simulink library "Display_THB3"  (Simulink 8.2)
settings: Solver=ode45  StartTime=0.0  StopTime=10.0  RelTol=1e-3
libraries: carnot x3
settings Model: Creator=lena.frank  LastModifiedBy=drhf

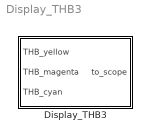
== system Display_THB3 ==
  Display_THB3 : Subsystem  mask(display THB){t=on, m=off, p=off, id=off, mix=off, d=off}
      mask prompts: t "temperature [degree centigrade]"; m "massflow [kg/s]"; p "pressure [Pa]"; id "fluid ID (1 = water, 2 = air, 3 = cotton oil, 4 = water-glycol)"; mix "fluid mix"; d "diameter [m]"
      mask help: Displays the ticked values from four THB.
      mask init:
      | v=[];
      | if (t)
      |     v  = [2];
      | end
      | if (m)
      |     v= [v 3];
      | end
      | if (p)
      |     v = [v 4];
      | end
      | if (id)
      |     v = [v 5];
      | end
      | if (mix)
      |     v = [v 6];
      | end
      | if (d)
      |     v = [v 7];
      | end
      mask Help: web(fullfile(path_carnot('help'),'display_THB.html'),'-helpbrowser')

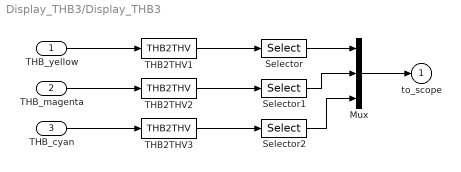
== system Display_THB3/Display_THB3 ==
  THB_yellow : Inport
  THB_magenta : Inport  Port=2
  THB_cyan : Inport  Port=3
  Mux : Mux  Inputs=3
  Selector : Selector  InputPortWidth=20  IndexOptions=Index vector (dialog)  Indices=[v]  OutputSizes=1
  Selector1 : Selector  InputPortWidth=20  IndexOptions=Index vector (dialog)  Indices=[v]  OutputSizes=1
  Selector2 : Selector  InputPortWidth=20  IndexOptions=Index vector (dialog)  Indices=[v]  OutputSizes=1
  THB2THV1 : carnot/Toolbox/THB2THV
  THB2THV2 : carnot/Toolbox/THB2THV
  THB2THV3 : carnot/Toolbox/THB2THV
  to_scope : Outport
  wires:
  Selector2/1 -> Mux/3
  THB_cyan/1 -> THB2THV3/1
  Selector1/1 -> Mux/2
  Mux/1 -> to_scope/1
  THB_magenta/1 -> THB2THV2/1
  Selector/1 -> Mux/1
  THB_yellow/1 -> THB2THV1/1
  THB2THV1/1 -> Selector/1
  THB2THV2/1 -> Selector1/1
  THB2THV3/1 -> Selector2/1
